simulink model "EX_Bus_Creator_1"  (Simulink 4.00)
settings: Solver=ode45  StartTime=0.0  StopTime=10.0  RelTol=1e-3

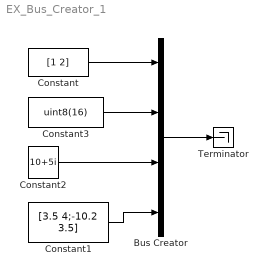
== system EX_Bus_Creator_1 ==
  Bus Creator : BusCreator  Inputs=4
  Constant : Constant  Value=[1 2]
  Constant1 : Constant  Value=[3.5 4;-10.2 3.5]  VectorParams1D=off
  Constant2 : Constant  Value=10+5i
  Constant3 : Constant  Value=uint8(16)
  Terminator : Terminator
  wires:
  Bus Creator/1 -> Terminator/1
  Constant3/1 -> Bus Creator/2
  Constant2/1 -> Bus Creator/3
  Constant/1 -> Bus Creator/1
  Constant1/1 -> Bus Creator/4
